simulink model "Part_3_Large_signal_model_without_controller"  (R2023b)
settings: Solver=ode4  StartTime=0.0  StopTime=10.0  FixedStep=0.0001  RelTol=1e-3
values from neighbouring files (symbols this model uses):
  J = 0.02    [Part_1_Solving_for_operating_points.m]
  Lr = 0.005974 + M    (= 0.311524)    [Part_1_Solving_for_operating_points.m]
  M = 0.30555    [Part_1_Solving_for_operating_points.m]
  np = 2    [Part_1_Solving_for_operating_points.m]
  Rr = 1 + 038 * 10^-3    (= 1.038)    [Part_1_Solving_for_operating_points.m]
  Rs = 1 + 300 * 10^-3    (= 1.3)    [Part_1_Solving_for_operating_points.m]
  sigma = (Ls *Lr - M^2)/(Lr)    (= 0.0118334384381)    [Part_1_Solving_for_operating_points.m]
settings Model: Creator=Santhosh  LastModifiedBy=Santhosh

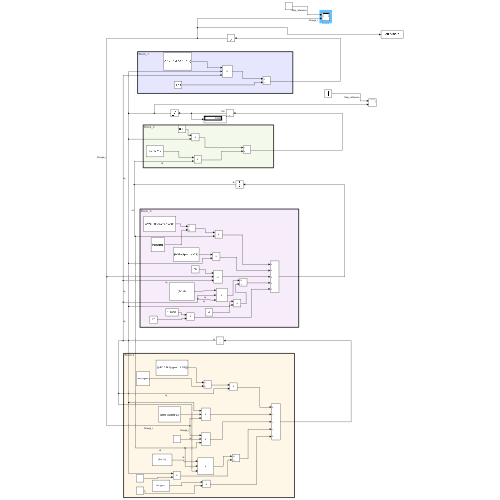
[thumbnail: Simulink's stored preview of the top-level diagram]
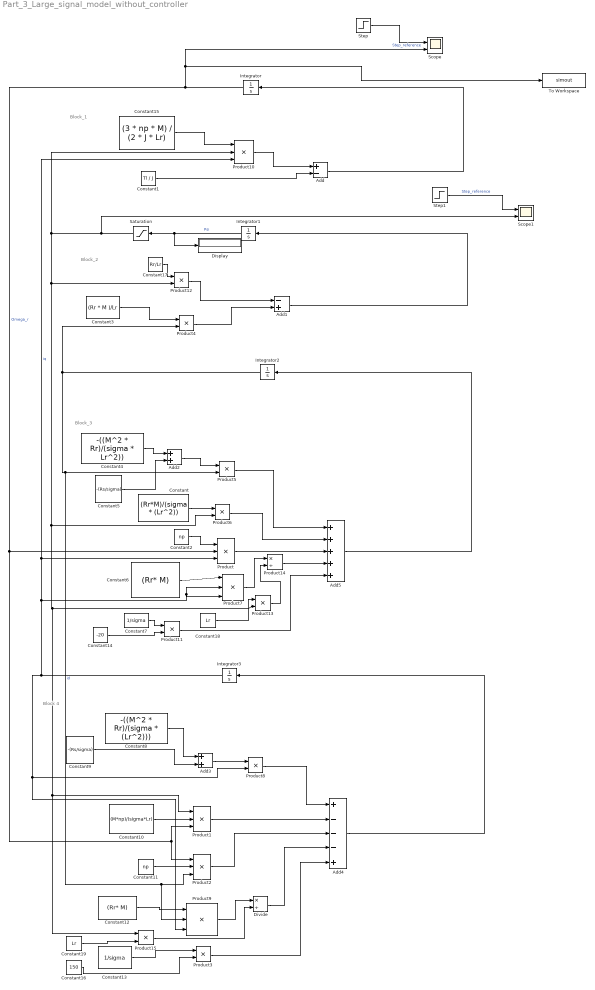
== system Part_3_Large_signal_model_without_controller ==
  note: Block_1
  note: Block_2
  note: Block_3
  note: Block 4
  Add : Sum  Inputs=+-
  Add1 : Sum  Inputs=-+
  Add2 : Sum
  Add3 : Sum
  Add4 : Sum  Inputs=+---+
  Add5 : Sum  Inputs=5
  Constant : Constant  Value=(Rr*M)/(sigma * (Lr^2))
  Constant1 : Constant  Value=Tl / J
  Constant10 : Constant  Value=(M*np)/(sigma*Lr)
  Constant11 : Constant  Value=np
  Constant12 : Constant  Value=(Rr* M)
  Constant13 : Constant  Value=1/sigma
  Constant14 : Constant  Value=-20
  Constant15 : Constant  Value=(3 * np * M) / (2 * J * Lr)
  Constant16 : Constant  Value=150
  Constant17 : Constant  Value=Rr/Lr
  Constant18 : Constant  Value=Lr
  Constant19 : Constant  Value=Lr
  Constant2 : Constant  Value=np
  Constant3 : Constant  Value=(Rr * M )/Lr
  Constant4 : Constant  Value=-((M^2 * Rr)/(sigma * Lr^2))
  Constant5 : Constant  Value=-(Rs/sigma)
  Constant6 : Constant  Value=(Rr* M)
  Constant7 : Constant  Value=1/sigma
  Constant8 : Constant  Value=-((M^2 * Rr)/(sigma * (Lr^2)))
  Constant9 : Constant  Value=-(Rs/sigma)
  Display : Display
  Divide : Product  Inputs=*/
  Integrator{,1..3} (4 alike) : Integrator
  Product{,1..2,10} (4 alike) : Product  Inputs=3
  Product{3..6,8,11..13,15} (9 alike) : Product
  Product14 : Product  Inputs=*/
  Product7 : Product  Inputs=***
  Product9 : Product  Inputs=***
  Saturation : Saturate  UpperLimit=1  LowerLimit=0.0001
  Scope : Scope  NumInputPorts=2
  Scope1 : Scope  NumInputPorts=2
  Step : Step  After=187.7  SampleTime=0
  Step1 : Step  After=0.36  SampleTime=0
  To Workspace : ToWorkspace  VariableName=simout  SaveFormat=Timeseries  SampleTime=-1
  wires:
  Add4/1 -> Integrator3/1
  Constant12/1 -> Product9/1
  Constant16/1 -> Product3/2
  Product8/1 -> Add4/1
  Constant8/1 -> Add3/1
  Product1/1 -> Add4/2
  Add3/1 -> Product8/1
  Constant9/1 -> Add3/2
  Constant13/1 -> Product3/1
  Product3/1 -> Add4/5
  Constant10/1 -> Product1/2
  Constant11/1 -> Product2/2
  Product2/1 -> Add4/3
  Product6/1 -> Add5/2
  Add2/1 -> Product5/1
  Product11/1 -> Add5/5
  Constant7/1 -> Product11/1
  Constant/1 -> Product6/1
  Constant6/1 -> Product7/1
  Product5/1 -> Add5/1
  Constant4/1 -> Add2/1
  Constant2/1 -> Product/1
  Product/1 -> Add5/3
  Add5/1 -> Integrator2/1
  Constant5/1 -> Add2/2
  Product4/1 -> Add1/2
  Product12/1 -> Add1/1
  Constant3/1 -> Product4/1
  Add1/1 -> Integrator1/1
  Constant15/1 -> Product10/1
  Constant1/1 -> Add/2
  Add/1 -> Integrator/1
  Product10/1 -> Add/1
  Constant14/1 -> Product11/2
  Integrator/1 -> To Workspace/1, Scope/2, Product2/1, Product1/3, Product/2  "Omega_r"
  Integrator1/1 -> Display/1, Saturation/1  "Psi"
  Integrator2/1 -> Product9/2, Product2/3, Product5/2, Product4/2  "id"
  Integrator3/1 -> Product9/3, Product8/2, Product7/2, Product7/3, Product/3, Product10/3  "iq"
  Product9/1 -> Divide/1
  Constant17/1 -> Product12/1
  Divide/1 -> Add4/4
  Constant18/1 -> Product13/1
  Product7/1 -> Product14/1
  Product13/1 -> Product14/2
  Product14/1 -> Add5/4
  Constant19/1 -> Product15/2
  Product15/1 -> Divide/2
  Saturation/1 -> Scope1/2, Product10/2, Product12/2, Product15/1, Product1/1, Product13/2, Product6/2
  Step/1 -> Scope/1  "Step_reference"
  Step1/1 -> Scope1/1  "Step_reference"
